simulink model "ctrl_student_HIL_DP"  (R2015a)
settings: Solver=ode3  StartTime=0.0  StopTime=10  FixedStep=0.01  RelTol=1e-3
values from neighbouring files (symbols this model uses):
  K2 = diag([200,50,3])    [Input_v3.m]    (also in inputDPgains.m = [1 0 0; 0 1 0; 0 0 1])
undefined symbols (not defined in the file or in its folder): L1, L2, L3
libraries: dspstat3 x1, simulink x1
(part 3 of 3)

== system ctrl_student_HIL_DP/Noise generator/noise generator/Band-limited white noise x ==
  step size : Inport
  power : Inport  Port=2
  Divide : Product  Inputs=*/
  Product : Product
  Sqrt : Sqrt  SaturateOnIntegerOverflow=on
  White Noise : RandomNumber  DisableCoverage=on  Seed=9024
  noise : Outport
  wires:
  White Noise/1 -> Product/2
  Product/1 -> noise/1
  step size/1 -> Divide/2
  Divide/1 -> Sqrt/1
  Sqrt/1 -> Product/1
  power/1 -> Divide/1

== system ctrl_student_HIL_DP/Noise generator/noise generator/Band-limited white noise y ==
  step size : Inport
  power : Inport  Port=2
  Divide : Product  Inputs=*/
  Product : Product
  Sqrt : Sqrt  SaturateOnIntegerOverflow=on
  White Noise : RandomNumber  DisableCoverage=on  Seed=123
  noise : Outport
  wires:
  White Noise/1 -> Product/2
  Product/1 -> noise/1
  step size/1 -> Divide/2
  Divide/1 -> Sqrt/1
  Sqrt/1 -> Product/1
  power/1 -> Divide/1

== matlab function ctrl_student_HIL_DP/joystick/Contoller_Map ==
  data: current_mode input; PosXLeft input; PosYLeft input; R2 input; tau_x output; tau_y output; tau_yaw output; glob_forces input
function [tau_x,tau_y,tau_yaw] = fcn(current_mode,PosXLeft,PosYLeft,R2,glob_forces)

if current_mode==2
    tau_x=-PosYLeft*glob_forces(1);
    tau_y=0;
    tau_yaw=PosXLeft*glob_forces(3); 
else
    tau_x=-PosYLeft*glob_forces(1);
    tau_y=PosXLeft*glob_forces(2);
    tau_yaw=R2*glob_forces(3);
end

end

== matlab function ctrl_student_HIL_DP/joystick/Force Allocation ==
  data: current_mode input; tau_x input; f_vspx output; tau_y input; tau_yaw input; f_vspy output; f_bt output
function [f_vspx,f_vspy,f_bt] = fcn(current_mode,tau_x,tau_y,tau_yaw)
l_bt=0.3875;
l_vsp=-0.4575;

if current_mode==2
    f_vspx=tau_x;
    f_vspy=0;
    f_bt=tau_y;
else
    %new equations from Silas 31/1/2017, based on Matlab inversion of B matrix
    f_vspx=tau_x;
    f_vspy=(l_bt*tau_y)/(l_bt - l_vsp) - tau_yaw/(l_bt - l_vsp);
    f_bt=tau_yaw/(l_bt - l_vsp) - (l_vsp*tau_y)/(l_bt - l_vsp);
end

%original equations from 30/1/2017
% f_vspx=tau_x;
% f_vspy=(tau_yaw-tau_y*l_bt)/(l_vsp-l_bt);
% f_bt=tau_y-f_vspy;

%tau_yaw = f_vspy*l_vsp+f_bt*l_bt
%tau_y=f_vspy+f_bt
%solve for f_bt and f_vspy




end

== matlab function ctrl_student_HIL_DP/Noise generator/Downsample	signal/MATLAB Function ==
  data: f input; h input; i input; count output
function count = fcn(f,h,i)
%#codegen
sampling_time = 1/f;
if (i+1)*h >= sampling_time
    count = 0;
else
    count = i+1;
end

== matlab function ctrl_student_HIL_DP/joystick/Force2Control ==
  data: f_vspx input; u_vsp output; f_vspy input; f_bt input; alpha output; u_bt output; sat_forces input
function [u_vsp,alpha,u_bt]   = fcn(f_vspx,f_vspy,f_bt,sat_forces)

u_vsp=sqrt(f_vspx^2+f_vspy^2)/sat_forces(1);
u_bt=f_bt/sat_forces(2);
alpha=atan2(f_vspy,f_vspx); 


end

== matlab function ctrl_student_HIL_DP/Noise generator/Sample & hold/MATLAB Function1 ==
  data: counter input; input input; hold input; output output
function output = fcn(counter,input,hold)
%#codegen

if counter == 0
    output = input;
else
    output = hold;
end

== matlab function ctrl_student_HIL_DP/joystick/Sat_Chk_BT ==
  data: u_inn input; u_out output; error output
function [u_out, error]= fcn(u_inn)

if u_inn > 1 || u_inn <-1
    u_out=0;
    error=true;
else
    u_out=u_inn;
    error=false;

end

== matlab function ctrl_student_HIL_DP/joystick/Sat_Chk_VSP ==
  data: u_inn input; u_out output; error output
function [u_out, error]= fcn(u_inn)

if u_inn > 1 || u_inn <-1
    u_out=0;
    error=true;
else
    u_out=u_inn;
    error=false;

end

== matlab function ctrl_student_HIL_DP/joystick/Sel_Control_Mode ==
  data: previous_condition input; select input; current_mode output
function current_mode= fcn(previous_condition, select)

if select==1
    if previous_condition ==2
        current_mode=3;
    else
        current_mode=2;
    end
else
    current_mode=previous_condition;
end

end

== matlab function ctrl_student_HIL_DP/DropOut_detector/dropoutDetect ==
  data: etaPrev input; eta input; dropout output; etaOut output
function [dropout,etaOut]= fcn(etaPrev,eta)

etaTemp=[etaPrev [eta; 0]];

if max(etaTemp(:,4))==1
     dropout=1;
elseif min(eta-etaTemp(1:3,end-1))==0
    dropout=1;
    etaTemp(4,end)=1;
elseif var(etaTemp(1,:))==0 || var(etaTemp(2,:))==0 || var(etaTemp(2,:))==0
    dropout=1;
else
    dropout=0;
end

etaOut=etaTemp(:,2:end);

end

== matlab function ctrl_student_HIL_DP/DropoutAction/accInjection ==
  data: uLast input; dropout input; uIn input; u_hat output; dVel input
function u_hat=accInj(uLast,dropout,uIn,dVel)

if dropout==false
    u_hat=uIn;
else
    u_hat=uLast+dVel;
end

== matlab function ctrl_student_HIL_DP/DPObserver/Bias/bHatDot ==
  data: bHatDot output; L3 input; eta input; etaHat input
function bHatDot = fcn(L3,eta,etaHat)

bHatDot=L3*(eta-etaHat);

end

== matlab function ctrl_student_HIL_DP/DPObserver/D ==
  data: D output; etaHatDot input
function D = fcn(etaHatDot)

u=0; %etaHatDot(1,1);
v=0; %etaHatDot(2,2);
r=0; %etaHatDot(3,3);

Xu=-0.6555;
Xuu=0.3545;
Xuuu=-3.787;
Yv=-1.33;
Yvv=-2.776;
Yvvv=-64.91;
Yr=-7.25;
Yrr=-3.45;
Yrrr=0;
Yrv=-0.805;
Yvr=-0.845;
Nv=0;
Nvv=-0.2088;
Nvvv=0;
Nr=-1.9;
Nrr=-0.75;
Nrrr=0;
Nrv=0.13;
Nvr=0.08;

d11=-Xu-Xuu*abs(u)-Xuuu*u^2;
d22=-Yv-Yvv*abs(v)-Yvvv*v^2-Yrv*abs(r);
d23=-Yr-Yvr*abs(v)-Yrr*abs(r)-Yrrr*r^2;
d32=-Nv-Nvv*abs(v)-Nvvv*v^2-Nrv*abs(r);
d33=-Nr-Nvr*abs(v)-Nrr*abs(r)-Nrrr*r^2;

D=[d11 0 0; 0 d22 d23; 0 d32 d33];

end

== matlab function ctrl_student_HIL_DP/DPObserver/Subsystem/M ==
  data: M output
function M = void

m=14.79;
M=[m+2 0 0; 0 m+10 m*0.0375; 0 m*0.0375 1.76+1];

end

== matlab function ctrl_student_HIL_DP/DPObserver/Subsystem/nuHatDot ==
  data: nuHat input; bHat input; D input; M input; K2 input; L2 input; tau input; eta input; R input; etaHat input; nuHatDot output
function nuHatDot = fcn(nuHat,bHat,D,M,K2,L2,tau,eta,R,etaHat)

nuHatDot=inv(M)*(-D*nuHat+transpose(R)*bHat+tau+K2*transpose(R)*L2*(eta-etaHat));

end

== matlab function ctrl_student_HIL_DP/DPObserver/calcR(psi)  ==
  data: psi input; R output
function R = fcn(psi)

R=[cos(psi) -sin(psi) 0; sin(psi) cos(psi) 0; 0 0 1];

end

== matlab function ctrl_student_HIL_DP/DPObserver/etaHat/etaHatDot ==
  data: etaHat input; nuHat input; L1 input; eta input; R input; etaHatDot output
function etaHatDot = fcn(etaHat,nuHat,L1,eta,R)

%etaHatDot=zeros(3,1);
etaHatDot=R*nuHat+L1*(eta-etaHat);

end
